simulink model "Module_Testing"  (R2023a)
settings: Solver=VariableStepAuto  StartTime=0.0  StopTime=10.0  RelTol=1e-3
undefined symbols (not defined in the file or in its folder): Drive_Motor_Control_D, Drive_Motor_Control_D_FilterCoeff, Drive_Motor_Control_D_LL, Drive_Motor_Control_D_UL, Drive_Motor_Control_FF, Drive_Motor_Control_I, Drive_Motor_Control_I_LL, Drive_Motor_Control_I_UL, Drive_Motor_Control_P, Steering_Motor_Control_D, Steering_Motor_Control_D_FilterCoeff, Steering_Motor_Control_D_LL, Steering_Motor_Control_D_UL, Steering_Motor_Control_I, Steering_Motor_Control_I_LL, Steering_Motor_Control_I_UL, Steering_Motor_Control_P, Swerve_Drive_lib, Swerve_Drive_Module, t_sample
libraries: Math x6, simulink x5, Simulation_lib x2, sm_lib x2, nesl_utility x1
settings Model: Creator=FIRSTMentor  LastModifiedBy=FIRSTMentor

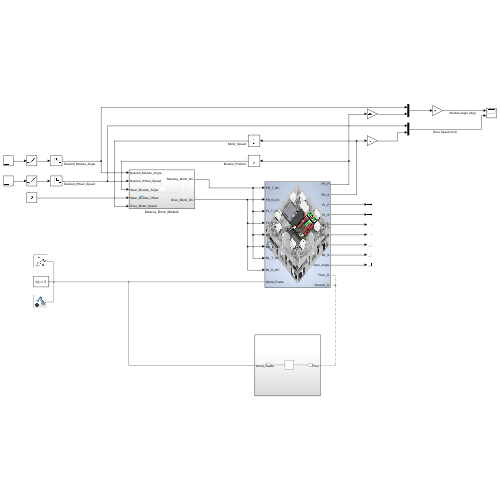
[thumbnail: Simulink's stored preview of the top-level diagram]
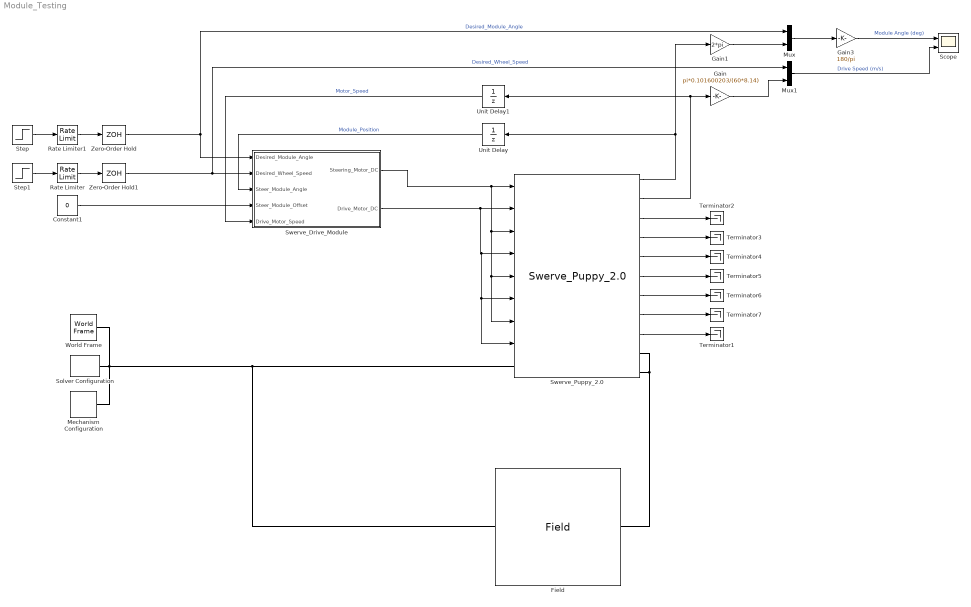
== system Module_Testing ==
  Constant1 : Constant  Value=0  SampleTime=t_sample
  Field : Simulation_lib/Field  SystemSampleTime=-1  VariantActivationTime=update diagram  Latency=0  AutoFrameSizeCalculation=off
  Gain : Gain  Gain=pi*0.101600203/(60*8.14)
  Gain1 : Gain  Gain=2*pi
  Gain3 : Gain  Gain=180/pi
  Mechanism Configuration : sm_lib/Utilities/Mechanism Configuration  UniformGravity=Constant  GravityVector=[0 0 -9.81]  GravityVectorUnits=m/s^2  LinearizationDelta=0.001  JointModeTransitionNonlinearIterations=2
  Mux : Mux  Inputs=2
  Mux1 : Mux  Inputs=2
  Rate Limiter : RateLimiter  RisingSlewLimit=3/0.5  FallingSlewLimit=-3/0.5  SampleTimeMode=inherited
  Rate Limiter1 : RateLimiter  RisingSlewLimit=(pi/2/0.5)  FallingSlewLimit=-(pi/2/0.5)  SampleTimeMode=inherited
  Scope : Scope  NumInputPorts=2
  Solver Configuration : nesl_utility/Solver Configuration  PhysicalDomain=network_engine_domain  SubClassName=solver  LeftPortType=input  RightPortType=generic  Tones=[]  Harmonics=[]  SimulateNoise=off  Profile=off  UseLocalSampling=off  EnableSwitchedLinearOptims=on  FrequencyDomain=off  UseCCode=off  RelTol=0.001  AbsTol=0.001  MinStep=1e-09  ToWorkspace=off  RevertToSquareIcSolve=off  NumHomotopyIterations=100  PhasorMode=off  PhasorModeNumHarmonics=1  ConsistencySolver=NEWTON_XTOL_AFTER_FTOL  IndexReductionMethod=DerivativeReplacement  DoDC=off  ResidualTolerance=1e-09  ConsistencyTolSource=GLOBAL  ConsistencyAbsTol=0.001  ConsistencyRelTol=0.001  ConsistencyTolFactor=0.001  UseLocalSolver=off  LocalSolverChoice=NE_BACKWARD_EULER_ADVANCER  ResolveIndetEquations=on  FunctionEvalNumThread=1  LocalSolverSampleTime=0.001  DoFixedCost=off  MaxNonlinIter=3  MaxModeIter=2  ComputeImpulses=off  ImpulseIterations=2  LinearAlgebra=auto  LinearAlgebraNumThread=0  EquationFormulation=NE_TIME_EF  DelaysMemoryBudget=1024  AutomaticFiltering=on  FilteringTimeConstant=0.001  PartitionStorageMethod=AS_NEEDED  PartitionMemoryBudget=1024  PartitionMethod=ROBUST
  Step : Step  Time=5  After=pi/2  SampleTime=t_sample
  Step1 : Step  After=3  SampleTime=t_sample
  Swerve_Drive_Module : Subsystem  AncestorBlock=Swerve_Drive_lib/Swerve_Drive_Module
      settings: LibrarySourceBlock=Swerve_Drive_lib/Swerve_Drive_Module
  Swerve_Puppy_2.0 : Simulation_lib/Swerve_Puppy_2.0  SystemSampleTime=-1  VariantActivationTime=update diagram  Latency=0  AutoFrameSizeCalculation=off
  Terminator{1..7} (7 alike) : Terminator
  Unit Delay : UnitDelay  SampleTime=t_sample  HasFrameUpgradeWarning=on
  Unit Delay1 : UnitDelay  SampleTime=t_sample  HasFrameUpgradeWarning=on
  World Frame : sm_lib/Frames and Transforms/World Frame
  Zero-Order Hold : ZeroOrderHold  SampleTime=t_sample
  Zero-Order Hold1 : ZeroOrderHold  SampleTime=t_sample
  wires:
  Swerve_Drive_Module/2(Drive_Motor_DC) -> Swerve_Puppy_2.0/2, Swerve_Puppy_2.0/4, Swerve_Puppy_2.0/8, Swerve_Puppy_2.0/6
  Swerve_Drive_Module/1(Steering_Motor_DC) -> Swerve_Puppy_2.0/1, Swerve_Puppy_2.0/3, Swerve_Puppy_2.0/7, Swerve_Puppy_2.0/5
  Swerve_Puppy_2.0/1 -> Gain1/1, Unit Delay/1
  Unit Delay/1 -> Swerve_Drive_Module/3(Steer_Module_Angle)  "Module_Position"
  Unit Delay1/1 -> Swerve_Drive_Module/5(Drive_Motor_Speed)  "Motor_Speed"
  Constant1/1 -> Swerve_Drive_Module/4(Steer_Module_Offset)
  Step/1 -> Rate Limiter1/1
  Step1/1 -> Rate Limiter/1
  Rate Limiter/1 -> Zero-Order Hold1/1
  Rate Limiter1/1 -> Zero-Order Hold/1
  Zero-Order Hold/1 -> Mux/1, Swerve_Drive_Module/1(Desired_Module_Angle)  "Desired_Module_Angle"
  Zero-Order Hold1/1 -> Mux1/1, Swerve_Drive_Module/2(Desired_Wheel_Speed)  "Desired_Wheel_Speed"
  Swerve_Puppy_2.0/2 -> Unit Delay1/1, Gain/1
  Mux/1 -> Gain3/1
  Mux1/1 -> Scope/2  "Drive Speed (m/s)"
  Gain/1 -> Mux1/2
  Gain1/1 -> Mux/2
  Gain3/1 -> Scope/1  "Module Angle (deg)"
  Swerve_Puppy_2.0/3 -> Terminator2/1
  Swerve_Puppy_2.0/4 -> Terminator3/1
  Swerve_Puppy_2.0/5 -> Terminator4/1
  Swerve_Puppy_2.0/6 -> Terminator5/1
  Swerve_Puppy_2.0/7 -> Terminator6/1
  Swerve_Puppy_2.0/8 -> Terminator7/1
  Swerve_Puppy_2.0/9 -> Terminator1/1
  connections:
  World Frame/RConn1 -- Mechanism Configuration/RConn1 -- Field/LConn1 -- Swerve_Puppy_2.0/LConn1 -- Solver Configuration/RConn1
  Field/RConn1 -- Swerve_Puppy_2.0/RConn1 -- Swerve_Puppy_2.0/RConn2

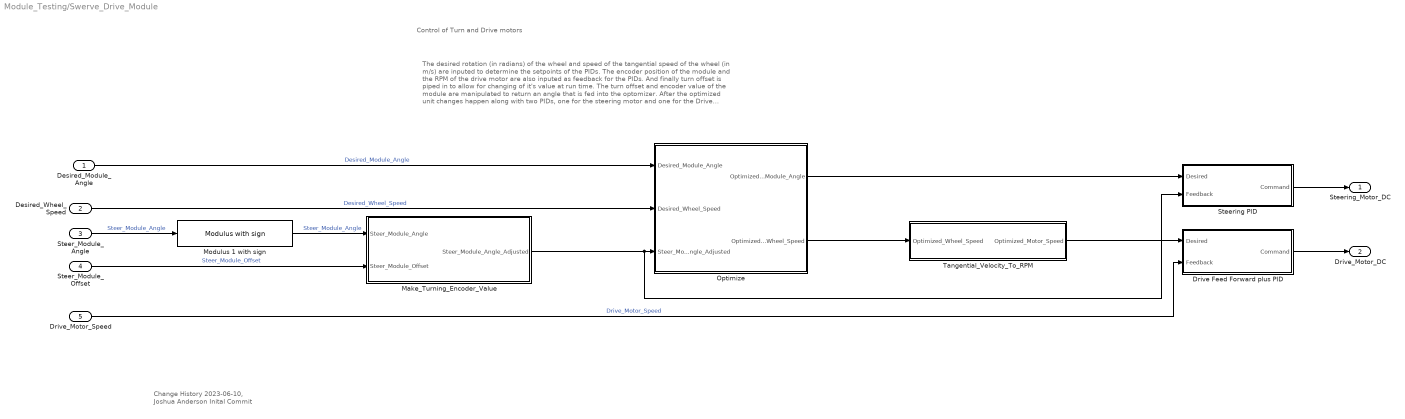
== system Module_Testing/Swerve_Drive_Module ==
  note: Control of Turn and Drive motors
  note: Change History
      | 2023-06-10, Joshua Anderson
      | Inital Commit
  note: The desired rotation (in radians) of the wheel and speed of the tangential speed of the wheel (in m/s) are inputed to determine the setpoints of the PIDs. The encoder position of the module and the RPM of the drive motor are also inputed as feedback for the PIDs. And finally turn offset is piped in to allow for changing of it's value at run time.
      | 	The turn offset and encoder value of the module are manipulated to return an angle that is fed into the optomizer. After the optimized unit changes happen along with two PIDs, one for the steering motor and one for the Drive motor.
  Desired_Module_Angle : Inport  OutDataTypeStr=double  Unit=rad
  Desired_Wheel_Speed : Inport  Port=2  OutDataTypeStr=double  Unit=m/s
  Steer_Module_Angle : Inport  Port=3  OutDataTypeStr=double  Unit=rev
  Steer_Module_Offset : Inport  Port=4  OutDataTypeStr=double  Unit=rev
  Drive_Motor_Speed : Inport  Port=5  OutDataTypeStr=double  Unit=rpm
  Drive Feed Forward plus PID : Subsystem  AncestorBlock=Math/Feed Forward plus PID  mask{Gain_FF=Drive_Motor_Control_FF, Gain_P=Drive_Motor_Control_P, Gain_I=Drive_Motor_Control_I, Gain_D=Drive_Motor_Control_D, FilterCoeff_D=Drive_Motor_Control_D_FilterCoeff, Limit_I_Upper=Drive_Motor_Control_I_UL, Limit_I_Lower=Drive_Motor_Control_I_LL, Limit_D_Upper=Drive_Motor_Control_D_UL, Limit_D_Lower=Drive_Motor_Control_D_LL, Limit_T_Upper=1, Limit_T_Lower=-1}
      mask prompts: Gain_FF "Feed Forward Gain"; Gain_P "Proportional Gain"; Gain_I "Integral Gain"; Gain_D "Derivative Gain"; FilterCoeff_D "Derivative Filter Coefficient"; Limit_I_Upper "Integral Upper Limit"; Limit_I_Lower "Integral Lower Limit"; Limit_D_Upper "Derivative Upper Limit"; Limit_D_Lower "Derivative Lower Limit"; Limit_T_Upper "Total Command Upper Limit"; Limit_T_Lower "Total Command Lower Limit"
      settings: LibrarySourceBlock=Math/Feed Forward plus PID
  Make_Turning_Encoder_Value : Subsystem
  Modulus 1 with sign : Math/Modulus with sign  Number=1
  Optimize : Subsystem
  Steering PID : Subsystem  AncestorBlock=Math/Feed Forward plus PID  mask{Gain_FF=0, Gain_P=Steering_Motor_Control_P, Gain_I=Steering_Motor_Control_I, Gain_D=Steering_Motor_Control_D, FilterCoeff_D=Steering_Motor_Control_D_FilterCoeff, Limit_I_Upper=Steering_Motor_Control_I_UL, Limit_I_Lower=Steering_Motor_Control_I_LL, Limit_D_Upper=Steering_Motor_Control_D_UL, Limit_D_Lower=Steering_Motor_Control_D_LL, Limit_T_Upper=1, Limit_T_Lower=-1}
      mask prompts: Gain_FF "Feed Forward Gain"; Gain_P "Proportional Gain"; Gain_I "Integral Gain"; Gain_D "Derivative Gain"; FilterCoeff_D "Derivative Filter Coefficient"; Limit_I_Upper "Integral Upper Limit"; Limit_I_Lower "Integral Lower Limit"; Limit_D_Upper "Derivative Upper Limit"; Limit_D_Lower "Derivative Lower Limit"; Limit_T_Upper "Total Command Upper Limit"; Limit_T_Lower "Total Command Lower Limit"
      settings: LibrarySourceBlock=Math/Feed Forward plus PID
  Tangential_Velocity_To_RPM : Subsystem
  Steering_Motor_DC : Outport  OutDataTypeStr=double  Unit=1
  Drive_Motor_DC : Outport  Port=2  OutDataTypeStr=double  Unit=1
  wires:
  Drive Feed Forward plus PID/1(Command) -> Drive_Motor_DC/1
  Optimize/1(Optimized_Module_Angle) -> Steering PID/1(Desired)
  Steering PID/1(Command) -> Steering_Motor_DC/1
  Steer_Module_Offset/1 -> Make_Turning_Encoder_Value/2(Steer_Module_Offset)  "Steer_Module_Offset"
  Make_Turning_Encoder_Value/1(Steer_Module_Angle_Adjusted) -> Optimize/3(Steer_Module_Angle_Adjusted), Steering PID/2(Feedback)
  Steer_Module_Angle/1 -> Modulus 1 with sign/1  "Steer_Module_Angle"
  Tangential_Velocity_To_RPM/1(Optimized_Motor_Speed) -> Drive Feed Forward plus PID/1(Desired)
  Optimize/2(Optimized_Wheel_Speed) -> Tangential_Velocity_To_RPM/1(Optimized_Wheel_Speed)
  Desired_Wheel_Speed/1 -> Optimize/2(Desired_Wheel_Speed)  "Desired_Wheel_Speed"
  Modulus 1 with sign/1 -> Make_Turning_Encoder_Value/1(Steer_Module_Angle)  "Steer_Module_Angle"
  Desired_Module_Angle/1 -> Optimize/1(Desired_Module_Angle)  "Desired_Module_Angle"
  Drive_Motor_Speed/1 -> Drive Feed Forward plus PID/2(Feedback)  "Drive_Motor_Speed"

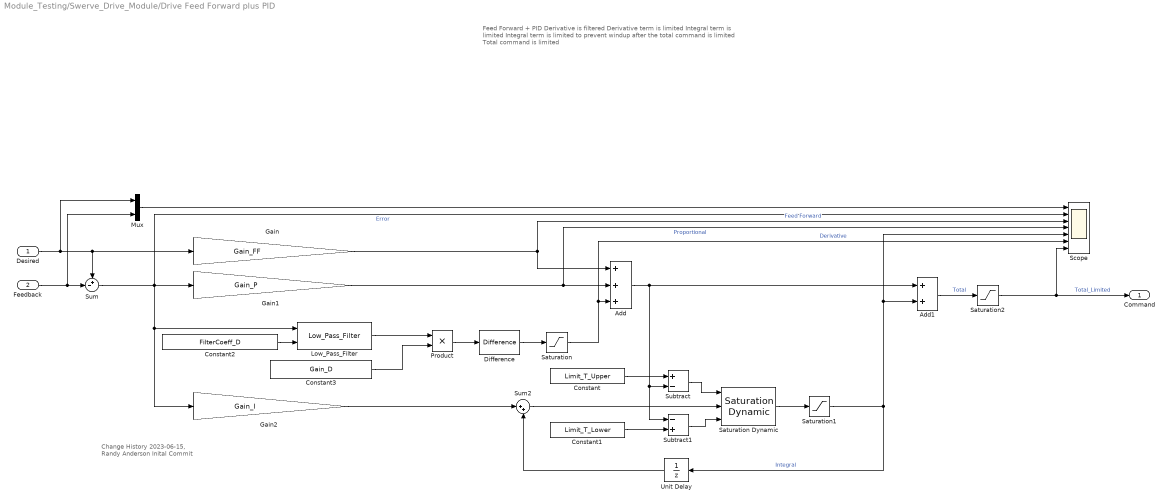
== system Module_Testing/Swerve_Drive_Module/Drive Feed Forward plus PID ==
  note: Change History
      | 2023-06-15, Randy Anderson
      | Inital Commit
  note: Feed Forward + PID
      |
      | Derivative is filtered
      | Derivative term is limited
      |
      | Integral term is limited
      |
      | Integral term is limited to prevent windup after the total command is limited
      |
      | Total command is limited
  Desired : Inport
  Feedback : Inport  Port=2
  Add : Sum  Inputs=3
  Add1 : Sum  Inputs=2
  Constant : Constant  Value=Limit_T_Upper
  Constant1 : Constant  Value=Limit_T_Lower
  Constant2 : Constant  Value=FilterCoeff_D
  Constant3 : Constant  Value=Gain_D
  Difference : simulink/Discrete/Difference  ICPrevInput=0.0  OutMin=[]  OutMax=[]  OutDataType=fixdt(1, 16)  OutScaling=2^-10  DoSatur=off
  Gain : Gain  Gain=Gain_FF
  Gain1 : Gain  Gain=Gain_P
  Gain2 : Gain  Gain=Gain_I
  Low_Pass_Filter : Math/Low_Pass_Filter  SystemSampleTime=-1  VariantActivationTime=update diagram  Latency=0  AutoFrameSizeCalculation=off
  Mux : Mux  Inputs=2
  Product : Product
  Saturation : Saturate  UpperLimit=Limit_D_Upper  LowerLimit=Limit_D_Lower
  Saturation Dynamic : simulink/Discontinuities/Saturation Dynamic  OutMin=[]  OutMax=[]  OutDataTypeStr=Inherit: Same as second input  OutDataType=fixdt(1, 16)  OutScaling=2^-10  DoSatur=off
  Saturation1 : Saturate  UpperLimit=Limit_I_Upper  LowerLimit=Limit_I_Lower
  Saturation2 : Saturate  UpperLimit=Limit_T_Upper  LowerLimit=Limit_T_Lower
  Scope : Scope  NumInputPorts=7
  Subtract : Sum  Inputs=+-
  Subtract1 : Sum  Inputs=-+
  Sum : Sum  Inputs=+-|
  Sum2 : Sum  Inputs=|++
  Unit Delay : UnitDelay  SampleTime=-1  HasFrameUpgradeWarning=on
  Command : Outport
  wires:
  Mux/1 -> Scope/1
  Saturation1/1 -> Add1/2, Scope/5, Unit Delay/1  "Integral"
  Saturation2/1 -> Command/1, Scope/7  "Total_Limited"
  Feedback/1 -> Sum/2, Mux/2
  Sum2/1 -> Saturation Dynamic/2
  Constant3/1 -> Product/2
  Constant2/1 -> Low_Pass_Filter/2
  Low_Pass_Filter/1 -> Product/1
  Product/1 -> Difference/1
  Saturation/1 -> Add/3, Scope/6  "Derivative"
  Difference/1 -> Saturation/1
  Desired/1 -> Gain/1, Sum/1, Mux/1
  Add1/1 -> Saturation2/1  "Total"
  Constant1/1 -> Subtract1/2
  Constant/1 -> Subtract/1
  Unit Delay/1 -> Sum2/2
  Subtract/1 -> Saturation Dynamic/1
  Saturation Dynamic/1 -> Saturation1/1
  Gain2/1 -> Sum2/1
  Gain1/1 -> Scope/4, Add/2  "Proportional"
  Subtract1/1 -> Saturation Dynamic/3
  Add/1 -> Subtract/2, Subtract1/1, Add1/1
  Gain/1 -> Scope/3, Add/1  "Feed Forward"
  Sum/1 -> Scope/2, Gain1/1, Low_Pass_Filter/1, Gain2/1  "Error"

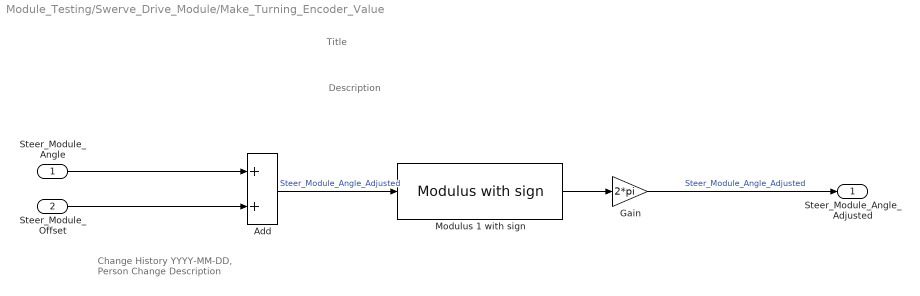
== system Module_Testing/Swerve_Drive_Module/Make_Turning_Encoder_Value ==
  note: Title
  note: Description
  note: Change History
      | YYYY-MM-DD, Person
      | Change Description
  Steer_Module_Angle : Inport  OutDataTypeStr=double  Unit=rev
  Steer_Module_Offset : Inport  Port=2  OutDataTypeStr=double  Unit=rev
  Add : Sum
  Gain : Gain  Gain=2*pi
  Modulus 1 with sign : Math/Modulus with sign  Number=1
  Steer_Module_Angle_Adjusted : Outport  OutDataTypeStr=double  Unit=rad
  wires:
  Modulus 1 with sign/1 -> Gain/1
  Gain/1 -> Steer_Module_Angle_Adjusted/1  "Steer_Module_Angle_Adjusted"
  Steer_Module_Angle/1 -> Add/1
  Steer_Module_Offset/1 -> Add/2
  Add/1 -> Modulus 1 with sign/1  "Steer_Module_Angle_Adjusted"

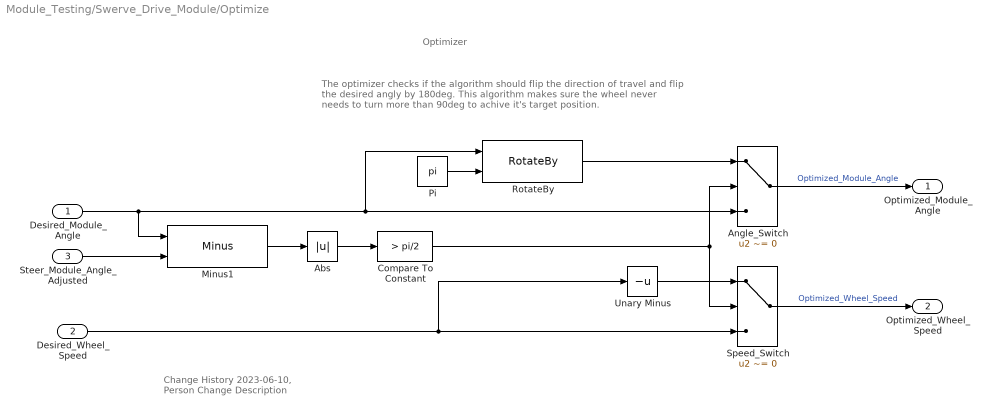
== system Module_Testing/Swerve_Drive_Module/Optimize ==
  note: Optimizer
  note: Change History
      | 2023-06-10, Person
      | Change Description
  note: The optimizer checks if the algorithm should flip the direction of travel and flip the desired angly by 180deg. This algorithm makes sure the wheel never needs to turn more than 90deg to achive it's target position.
  Desired_Module_Angle : Inport  OutDataTypeStr=double  Unit=rad
  Desired_Wheel_Speed : Inport  Port=2  OutDataTypeStr=double  Unit=m/s
  Steer_Module_Angle_Adjusted : Inport  Port=3  OutDataTypeStr=double  Unit=rad
  Abs : Abs  SaturateOnIntegerOverflow=off
  Angle_Switch : Switch  Criteria=u2 ~= 0  SaturateOnIntegerOverflow=off  InputSameDT=off
  Compare To Constant : simulink/Logic and Bit Operations/Compare To Constant  relop=>  const=pi/2  OutDataTypeStr=boolean
  Minus1 : Math/Minus  SystemSampleTime=-1  VariantActivationTime=update diagram  Latency=0  AutoFrameSizeCalculation=off
  Pi : Constant  Value=pi  OutDataTypeStr=Inherit: Inherit via back propagation
  RotateBy : Math/RotateBy  SystemSampleTime=-1  VariantActivationTime=update diagram  Latency=0  AutoFrameSizeCalculation=off
  Speed_Switch : Switch  Criteria=u2 ~= 0  SaturateOnIntegerOverflow=off  InputSameDT=off
  Unary Minus : UnaryMinus
  Optimized_Module_Angle : Outport  OutDataTypeStr=double  Unit=rad
  Optimized_Wheel_Speed : Outport  Port=2  OutDataTypeStr=double  Unit=m/s
  wires:
  RotateBy/1 -> Angle_Switch/1
  Speed_Switch/1 -> Optimized_Wheel_Speed/1  "Optimized_Wheel_Speed"
  Angle_Switch/1 -> Optimized_Module_Angle/1  "Optimized_Module_Angle"
  Pi/1 -> RotateBy/2
  Unary Minus/1 -> Speed_Switch/1
  Compare To Constant/1 -> Speed_Switch/2, Angle_Switch/2
  Desired_Wheel_Speed/1 -> Speed_Switch/3, Unary Minus/1
  Abs/1 -> Compare To Constant/1
  Minus1/1 -> Abs/1
  Steer_Module_Angle_Adjusted/1 -> Minus1/2
  Desired_Module_Angle/1 -> Angle_Switch/3, RotateBy/1, Minus1/1

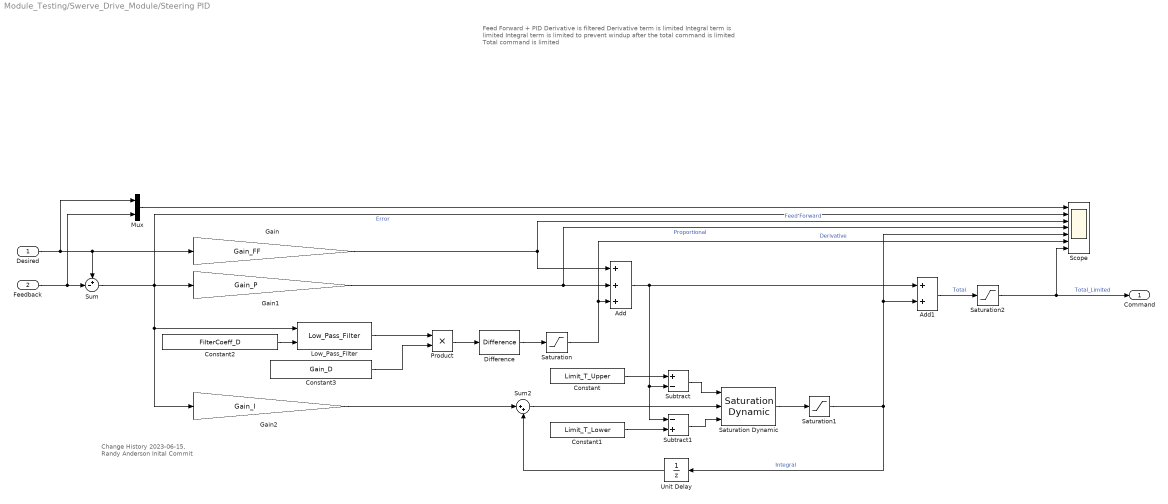
== system Module_Testing/Swerve_Drive_Module/Steering PID ==
  note: Change History
      | 2023-06-15, Randy Anderson
      | Inital Commit
  note: Feed Forward + PID
      |
      | Derivative is filtered
      | Derivative term is limited
      |
      | Integral term is limited
      |
      | Integral term is limited to prevent windup after the total command is limited
      |
      | Total command is limited
  Desired : Inport
  Feedback : Inport  Port=2
  Add : Sum  Inputs=3
  Add1 : Sum  Inputs=2
  Constant : Constant  Value=Limit_T_Upper
  Constant1 : Constant  Value=Limit_T_Lower
  Constant2 : Constant  Value=FilterCoeff_D
  Constant3 : Constant  Value=Gain_D
  Difference : simulink/Discrete/Difference  ICPrevInput=0.0  OutMin=[]  OutMax=[]  OutDataType=fixdt(1, 16)  OutScaling=2^-10  DoSatur=off
  Gain : Gain  Gain=Gain_FF
  Gain1 : Gain  Gain=Gain_P
  Gain2 : Gain  Gain=Gain_I
  Low_Pass_Filter : Math/Low_Pass_Filter  SystemSampleTime=-1  VariantActivationTime=update diagram  Latency=0  AutoFrameSizeCalculation=off
  Mux : Mux  Inputs=2
  Product : Product
  Saturation : Saturate  UpperLimit=Limit_D_Upper  LowerLimit=Limit_D_Lower
  Saturation Dynamic : simulink/Discontinuities/Saturation Dynamic  OutMin=[]  OutMax=[]  OutDataTypeStr=Inherit: Same as second input  OutDataType=fixdt(1, 16)  OutScaling=2^-10  DoSatur=off
  Saturation1 : Saturate  UpperLimit=Limit_I_Upper  LowerLimit=Limit_I_Lower
  Saturation2 : Saturate  UpperLimit=Limit_T_Upper  LowerLimit=Limit_T_Lower
  Scope : Scope  NumInputPorts=7
  Subtract : Sum  Inputs=+-
  Subtract1 : Sum  Inputs=-+
  Sum : Sum  Inputs=+-|
  Sum2 : Sum  Inputs=|++
  Unit Delay : UnitDelay  SampleTime=-1  HasFrameUpgradeWarning=on
  Command : Outport
  wires:
  Mux/1 -> Scope/1
  Saturation1/1 -> Add1/2, Scope/5, Unit Delay/1  "Integral"
  Saturation2/1 -> Command/1, Scope/7  "Total_Limited"
  Feedback/1 -> Sum/2, Mux/2
  Sum2/1 -> Saturation Dynamic/2
  Constant3/1 -> Product/2
  Constant2/1 -> Low_Pass_Filter/2
  Low_Pass_Filter/1 -> Product/1
  Product/1 -> Difference/1
  Saturation/1 -> Add/3, Scope/6  "Derivative"
  Difference/1 -> Saturation/1
  Desired/1 -> Gain/1, Sum/1, Mux/1
  Add1/1 -> Saturation2/1  "Total"
  Constant1/1 -> Subtract1/2
  Constant/1 -> Subtract/1
  Unit Delay/1 -> Sum2/2
  Subtract/1 -> Saturation Dynamic/1
  Saturation Dynamic/1 -> Saturation1/1
  Gain2/1 -> Sum2/1
  Gain1/1 -> Scope/4, Add/2  "Proportional"
  Subtract1/1 -> Saturation Dynamic/3
  Add/1 -> Subtract/2, Subtract1/1, Add1/1
  Gain/1 -> Scope/3, Add/1  "Feed Forward"
  Sum/1 -> Scope/2, Gain1/1, Low_Pass_Filter/1, Gain2/1  "Error"

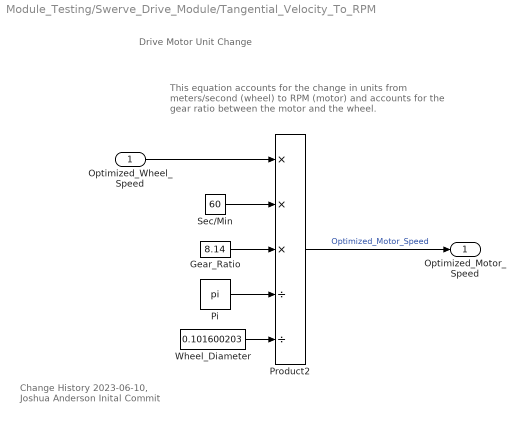
== system Module_Testing/Swerve_Drive_Module/Tangential_Velocity_To_RPM ==
  note: Drive Motor Unit Change
  note: Change History
      | 2023-06-10, Joshua Anderson
      | Inital Commit
  note: This equation accounts for the change in units from meters/second (wheel) to RPM (motor) and accounts for the gear ratio between the motor and the wheel.
  Optimized_Wheel_Speed : Inport  Unit=m/s
  Gear_Ratio : Constant  Value=8.14
  Pi : Constant  Value=pi  OutDataTypeStr=Inherit: Inherit via back propagation
  Product2 : Product  Inputs=***//
  Sec/Min : Constant  Value=60
  Wheel_Diameter : Constant  Value=0.101600203
  Optimized_Motor_Speed : Outport  Unit=rpm
  wires:
  Wheel_Diameter/1 -> Product2/5
  Pi/1 -> Product2/4
  Optimized_Wheel_Speed/1 -> Product2/1
  Product2/1 -> Optimized_Motor_Speed/1  "Optimized_Motor_Speed"
  Gear_Ratio/1 -> Product2/3
  Sec/Min/1 -> Product2/2
